simulink model "Merge_Tryout"  (R2020b)
settings: Solver=VariableStepAuto  StartTime=0.0  StopTime=60  RelTol=1e-3
values from neighbouring files (symbols this model uses):
  A_2 = zeros(3)    [MPC_tune.m]
  B_2 = I_inv    [MPC_tune.m]
  C_2 = eye(3)    [MPC_tune.m]
  D_2 = zeros(3)    [MPC_tune.m]
  I_inv = inv(I_mat)    [MPC_tune.m]
undefined symbols (not defined in the file or in its folder): theta0, x0
libraries: fuzblock x6, pid_lib x3, mpclib x2, dspmathops x2, dspsigops x2
settings Model: Creator=Jonathan van Zyl  LastModifiedBy=Jonathan van Zyl

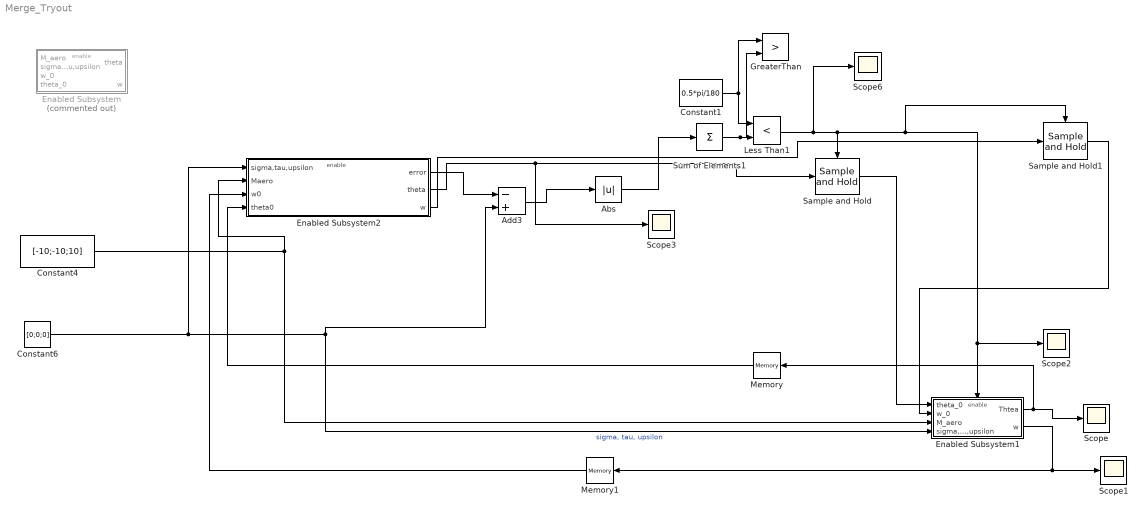
== system Merge_Tryout ==
  Abs : Abs
  Add3 : Sum  Inputs=-+
  Constant1 : Constant  Value=0.5*pi/180
  Constant4 : Constant  Value=[-10;-10;10]
  Constant6 : Constant  Value=[0;0;0]
  Enabled Subsystem : Subsystem  Commented=on  TreatAsAtomicUnit=on
  Enabled Subsystem1 : Subsystem  TreatAsAtomicUnit=on
  Enabled Subsystem2 : Subsystem  TreatAsAtomicUnit=on
  GreaterThan : RelationalOperator  Operator=>  OutDataTypeStr=boolean  RndMeth=Simplest
  Less Than1 : RelationalOperator  Operator=<  OutDataTypeStr=boolean  RndMeth=Simplest
  Memory : Memory
  Memory1 : Memory
  Sample and Hold : dspsigops/Sample and Hold  trig=Rising edge  initCond=0  latchinput=off
  Sample and Hold1 : dspsigops/Sample and Hold  trig=Rising edge  initCond=0  latchinput=off
  Scope{,1..3,6} (5 alike) : Scope
  Sum of Elements1 : Sum  Inputs=+
  wires:
  Constant4/1 -> Enabled Subsystem2/2(Maero), Enabled Subsystem1/3(M_aero)
  Constant6/1 -> Add3/2, Enabled Subsystem1/4(sigma,tau,upsilon), Enabled Subsystem2/1(sigma,tau,upsilon)  "sigma, tau, upsilon"
  Add3/1 -> Abs/1
  Less Than1/1 -> Scope2/1, Enabled Subsystem1/Enable, Sample and Hold1/Trigger, Sample and Hold/Trigger, Scope6/1
  Sum of Elements1/1 -> GreaterThan/2, Less Than1/2
  Constant1/1 -> GreaterThan/1, Less Than1/1
  Abs/1 -> Sum of Elements1/1
  Sample and Hold/1 -> Enabled Subsystem1/1(theta_0)
  Sample and Hold1/1 -> Enabled Subsystem1/2(w_0)
  Enabled Subsystem2/1(error) -> Add3/1
  ? -> Enabled Subsystem2/Enable
  Enabled Subsystem1/1(Thtea) -> Memory/1, Scope/1
  Enabled Subsystem2/2(theta) -> Scope3/1, Sample and Hold/1
  Enabled Subsystem2/3(w) -> Sample and Hold1/1
  Memory/1 -> Enabled Subsystem2/4(theta0)
  Enabled Subsystem1/2(w) -> Memory1/1, Scope1/1
  Memory1/1 -> Enabled Subsystem2/3(w0)

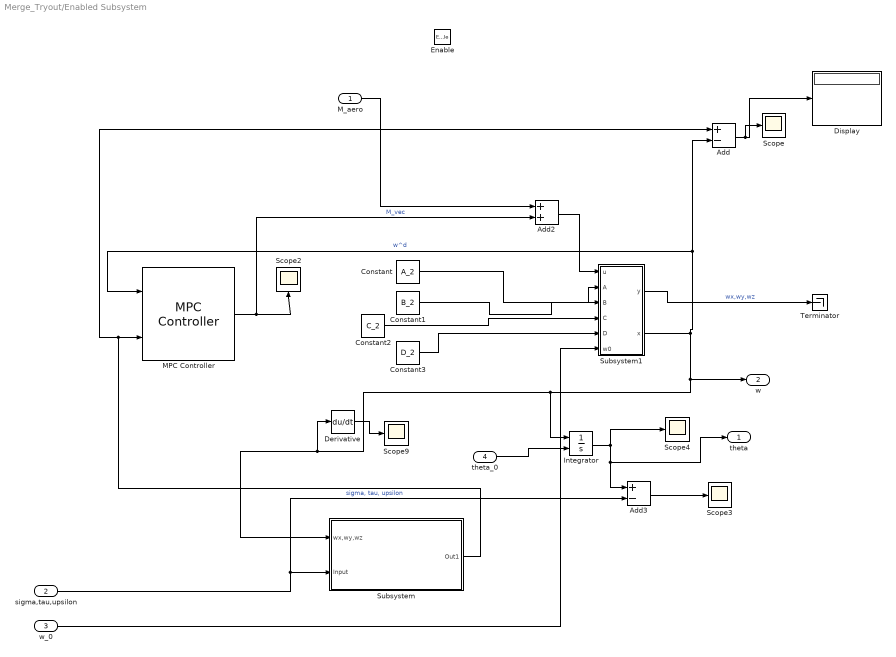
== system Merge_Tryout/Enabled Subsystem ==
  M_aero : Inport
  sigma,tau,upsilon : Inport  Port=2
  w_0 : Inport  Port=3
  theta_0 : Inport  Port=4
  Enable : EnablePort
  Add : Sum  Inputs=+-
  Add2 : Sum
  Add3 : Sum  Inputs=+-
  Constant : Constant  Value=A_2
  Constant1 : Constant  Value=B_2
  Constant2 : Constant  Value=C_2
  Constant3 : Constant  Value=D_2
  Derivative : Derivative
  Display : Display
  Integrator : Integrator  InitialConditionSource=external
  MPC Controller : mpclib/MPC Controller  SCDEnableBlockLinearizationSpecification=on  mpcobj=MPCDesignerSession.AppData.Controllers.MPC  is_multiple=0  enable_value=0  return_u0=off  updateMPCinCallerWorkspace=on  md_inport=off  mv_inport=off  uref_inport=off  return_cost=off  return_mvseq=off  return_qpstatus=off  return_xseq=off  return_state=off  return_ovseq=off  state_inport=off  umin_inport=off  umax_inport=off  ymin_inport=off  ymax_inport=off  cc_inport=off  ywt_inport=off  uwt_inport=off  duwt_inport=off  rhoeps_inport=off  pm_inport=off  MaximumP=10  HorizonChoice=FixedHorizon  n_ts=0.1  n_p=10  n_mv=3  n_md=0  n_ud=0  n_mo=3  n_uo=0  BlockDataType=double  SampleTimeInherited=off  switch_inport=off
  Scope{,2..4,9} (5 alike) : Scope
  Subsystem : Subsystem
  Subsystem1 : Subsystem
  Terminator : Terminator
  theta : Outport
  w : Outport  Port=2
  wires:
  Constant2/1 -> Subsystem1/4(C)
  Subsystem1/2(x) -> Add/2, MPC Controller/1, w/1, Integrator/1, Subsystem/1(wx,wy,wz), Derivative/1  "w^d"
  Derivative/1 -> Scope9/1
  MPC Controller/1 -> Add2/2, Scope2/1  "M_vec"
  Constant3/1 -> Subsystem1/5(D)
  sigma,tau,upsilon/1 -> Add3/2, Subsystem/2(Input)  "sigma, tau, upsilon"
  Subsystem/1(Out1) -> Add/1, MPC Controller/2
  M_aero/1 -> Add2/1
  Add/1 -> Display/1, Scope/1
  Constant/1 -> Subsystem1/2(A)
  Add2/1 -> Subsystem1/1(u)
  Add3/1 -> Scope3/1
  Subsystem1/1(y) -> Terminator/1  "wx,wy,wz"
  Constant1/1 -> Subsystem1/3(B)
  Integrator/1 -> Scope4/1, Add3/1, theta/1
  w_0/1 -> Subsystem1/6(w0)
  theta_0/1 -> Integrator/2

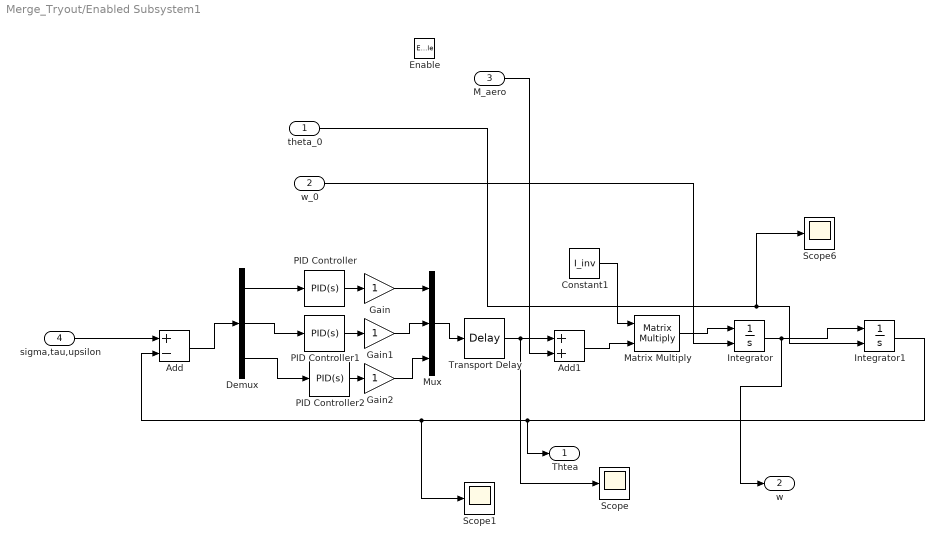
== system Merge_Tryout/Enabled Subsystem1 ==
  theta_0 : Inport
  w_0 : Inport  Port=2
  M_aero : Inport  Port=3
  sigma,tau,upsilon : Inport  Port=4
  Enable : EnablePort
  Add : Sum  Inputs=+-
  Add1 : Sum
  Constant1 : Constant  Value=I_inv
  Demux : Demux  Outputs=3
  Gain : Gain
  Gain1 : Gain
  Gain2 : Gain
  Integrator : Integrator  InitialConditionSource=external  InitialCondition=[0.15;-0.2;0.01]
  Integrator1 : Integrator  InitialConditionSource=external  InitialCondition=[0.01;-0.01;0.005]
  Matrix Multiply : Product  Multiplication=Matrix(*)
  Mux : Mux  Inputs=3
  PID Controller : pid_lib/PID Controller  Controller=PID  Form=Parallel  TimeDomain=Continuous-time  UseExternalTs=off  SampleTime=-1  IntegratorMethod=Forward Euler  FilterMethod=Forward Euler  ControllerParametersSource=internal  P=76.4274415550338  I=3.57793373088927  D=400.875615235633  UseFilter=on  N=5.45397025421619  TunerSelectOption=Transfer Function Based (PID Tuner App)  InitialConditionSource=internal  InitialConditionForIntegrator=0  InitialConditionForFilter=0  DifferentiatorICPrevScaledInput=0  ExternalReset=none  TrackingMode=off  Kt=1  LimitOutput=off  SatLimitsSource=internal  UpperSaturationLimit=inf  LowerSaturationLimit=-inf  LinearizeAsGain=on  AntiWindupMode=none  Kb=1  POutMin=[]  POutMax=[]  IOutMin=[]  IOutMax=[]  DOutMin=[]  DOutMax=[]  NOutMin=[]  NOutMax=[]  SumOutMin=[]  SumOutMax=[]  SaturationOutMin=[]  SaturationOutMax=[]  PParamMin=[]  PParamMax=[]  IParamMin=[]  IParamMax=[]  DParamMin=[]  DParamMax=[]  NParamMin=[]  NParamMax=[]  KbParamMin=[]  KbParamMax=[]  KtParamMin=[]  KtParamMax=[]  KbOutMin=[]  KbOutMax=[]  KtOutMin=[]  KtOutMax=[]  IntegratorOutMin=[]  IntegratorOutMax=[]  FilterOutMin=[]  FilterOutMax=[]  SumI1OutMin=[]  SumI1OutMax=[]  SumI2OutMin=[]  SumI2OutMax=[]  SumI3OutMin=[]  SumI3OutMax=[]  SumI4OutMin=[]  SumI4OutMax=[]  SumDOutMin=[]  SumDOutMax=[]  DifferentiatorOutMin=[]  DifferentiatorOutMax=[]  FilterDiffOutCoefMin=[]  FilterDiffOutCoefMax=[]  ReciprocalOutMin=[]  ReciprocalOutMax=[]  SumDenOutMin=[]  SumDenOutMax=[]  SumNumOutMin=[]  SumNumOutMax=[]  DivideOutMin=[]  DivideOutMax=[]  UdiffTsProdOutMin=[]  UdiffTsProdOutMax=[]  NTsProdOutMin=[]  NTsProdOutMax=[]  UintegralTsProdOutMin=[]  UintegralTsProdOutMax=[]  UngainTsProdOutMin=[]  UngainTsProdOutMax=[]  IntegratorContinuousStateAttributes=''  IntegratorStateMustResolveToSignalObject=off  IntegratorRTWStateStorageClass=Auto  FilterContinuousStateAttributes=''  FilterStateMustResolveToSignalObject=off  FilterRTWStateStorageClass=Auto  ParallelPVariant=InternalParameters  IdealPVariant=Disabled  IVariant=InternalParameters  DVariant=InternalParameters  IntegratorVariant=Continuous  SatVariant=Disabled  AWVariant=Passthrough  PCopyVariant=Disabled  TRVariant=Disabled  FdbkBlocksVariant=Forward  IdealPFdbkVariant=Disabled  SatFdbkVariant=Disabled  DerivativeFilterVariant=ContFilter  NVariant=InternalParameters  NCopyVariant=Disabled  FilterICVariant=InternalICsFilter  IntegratorICVariant=InternalICs  ExternalResetVariant=Disabled  TRSumVariant=Passthrough  SumFdbkVariant=Disabled  SumVariant=Sum_PID  TsampFilterVariant=InternalTs  TsampNgainVariant=Passthrough  TsampIntegralVariant=Passthrough  ExternalSaturationOutDataTypeStr=Inherit: Same as second input
  PID Controller1 : pid_lib/PID Controller  Controller=PID  Form=Parallel  TimeDomain=Continuous-time  UseExternalTs=off  SampleTime=-1  IntegratorMethod=Forward Euler  FilterMethod=Forward Euler  ControllerParametersSource=internal  P=-202.527799620363  I=-9.48129403471772  D=-1062.29457146841  UseFilter=on  N=5.45397025421619  TunerSelectOption=Transfer Function Based (PID Tuner App)  InitialConditionSource=internal  InitialConditionForIntegrator=0  InitialConditionForFilter=0  DifferentiatorICPrevScaledInput=0  ExternalReset=none  TrackingMode=off  Kt=1  LimitOutput=off  SatLimitsSource=internal  UpperSaturationLimit=inf  LowerSaturationLimit=-inf  LinearizeAsGain=on  AntiWindupMode=none  Kb=1  POutMin=[]  POutMax=[]  IOutMin=[]  IOutMax=[]  DOutMin=[]  DOutMax=[]  NOutMin=[]  NOutMax=[]  SumOutMin=[]  SumOutMax=[]  SaturationOutMin=[]  SaturationOutMax=[]  PParamMin=[]  PParamMax=[]  IParamMin=[]  IParamMax=[]  DParamMin=[]  DParamMax=[]  NParamMin=[]  NParamMax=[]  KbParamMin=[]  KbParamMax=[]  KtParamMin=[]  KtParamMax=[]  KbOutMin=[]  KbOutMax=[]  KtOutMin=[]  KtOutMax=[]  IntegratorOutMin=[]  IntegratorOutMax=[]  FilterOutMin=[]  FilterOutMax=[]  SumI1OutMin=[]  SumI1OutMax=[]  SumI2OutMin=[]  SumI2OutMax=[]  SumI3OutMin=[]  SumI3OutMax=[]  SumI4OutMin=[]  SumI4OutMax=[]  SumDOutMin=[]  SumDOutMax=[]  DifferentiatorOutMin=[]  DifferentiatorOutMax=[]  FilterDiffOutCoefMin=[]  FilterDiffOutCoefMax=[]  ReciprocalOutMin=[]  ReciprocalOutMax=[]  SumDenOutMin=[]  SumDenOutMax=[]  SumNumOutMin=[]  SumNumOutMax=[]  DivideOutMin=[]  DivideOutMax=[]  UdiffTsProdOutMin=[]  UdiffTsProdOutMax=[]  NTsProdOutMin=[]  NTsProdOutMax=[]  UintegralTsProdOutMin=[]  UintegralTsProdOutMax=[]  UngainTsProdOutMin=[]  UngainTsProdOutMax=[]  IntegratorContinuousStateAttributes=''  IntegratorStateMustResolveToSignalObject=off  IntegratorRTWStateStorageClass=Auto  FilterContinuousStateAttributes=''  FilterStateMustResolveToSignalObject=off  FilterRTWStateStorageClass=Auto  ParallelPVariant=InternalParameters  IdealPVariant=Disabled  IVariant=InternalParameters  DVariant=InternalParameters  IntegratorVariant=Continuous  SatVariant=Disabled  AWVariant=Passthrough  PCopyVariant=Disabled  TRVariant=Disabled  FdbkBlocksVariant=Forward  IdealPFdbkVariant=Disabled  SatFdbkVariant=Disabled  DerivativeFilterVariant=ContFilter  NVariant=InternalParameters  NCopyVariant=Disabled  FilterICVariant=InternalICsFilter  IntegratorICVariant=InternalICs  ExternalResetVariant=Disabled  TRSumVariant=Passthrough  SumFdbkVariant=Disabled  SumVariant=Sum_PID  TsampFilterVariant=InternalTs  TsampNgainVariant=Passthrough  TsampIntegralVariant=Passthrough  ExternalSaturationOutDataTypeStr=Inherit: Same as second input
  PID Controller2 : pid_lib/PID Controller  Controller=PID  Form=Parallel  TimeDomain=Continuous-time  UseExternalTs=off  SampleTime=-1  IntegratorMethod=Forward Euler  FilterMethod=Forward Euler  ControllerParametersSource=internal  P=-232.294042315359  I=-10.8747940867059  D=-1218.42384402842  UseFilter=on  N=5.45397025421619  TunerSelectOption=Transfer Function Based (PID Tuner App)  InitialConditionSource=internal  InitialConditionForIntegrator=0  InitialConditionForFilter=0  DifferentiatorICPrevScaledInput=0  ExternalReset=none  TrackingMode=off  Kt=1  LimitOutput=off  SatLimitsSource=internal  UpperSaturationLimit=inf  LowerSaturationLimit=-inf  LinearizeAsGain=on  AntiWindupMode=none  Kb=1  POutMin=[]  POutMax=[]  IOutMin=[]  IOutMax=[]  DOutMin=[]  DOutMax=[]  NOutMin=[]  NOutMax=[]  SumOutMin=[]  SumOutMax=[]  SaturationOutMin=[]  SaturationOutMax=[]  PParamMin=[]  PParamMax=[]  IParamMin=[]  IParamMax=[]  DParamMin=[]  DParamMax=[]  NParamMin=[]  NParamMax=[]  KbParamMin=[]  KbParamMax=[]  KtParamMin=[]  KtParamMax=[]  KbOutMin=[]  KbOutMax=[]  KtOutMin=[]  KtOutMax=[]  IntegratorOutMin=[]  IntegratorOutMax=[]  FilterOutMin=[]  FilterOutMax=[]  SumI1OutMin=[]  SumI1OutMax=[]  SumI2OutMin=[]  SumI2OutMax=[]  SumI3OutMin=[]  SumI3OutMax=[]  SumI4OutMin=[]  SumI4OutMax=[]  SumDOutMin=[]  SumDOutMax=[]  DifferentiatorOutMin=[]  DifferentiatorOutMax=[]  FilterDiffOutCoefMin=[]  FilterDiffOutCoefMax=[]  ReciprocalOutMin=[]  ReciprocalOutMax=[]  SumDenOutMin=[]  SumDenOutMax=[]  SumNumOutMin=[]  SumNumOutMax=[]  DivideOutMin=[]  DivideOutMax=[]  UdiffTsProdOutMin=[]  UdiffTsProdOutMax=[]  NTsProdOutMin=[]  NTsProdOutMax=[]  UintegralTsProdOutMin=[]  UintegralTsProdOutMax=[]  UngainTsProdOutMin=[]  UngainTsProdOutMax=[]  IntegratorContinuousStateAttributes=''  IntegratorStateMustResolveToSignalObject=off  IntegratorRTWStateStorageClass=Auto  FilterContinuousStateAttributes=''  FilterStateMustResolveToSignalObject=off  FilterRTWStateStorageClass=Auto  ParallelPVariant=InternalParameters  IdealPVariant=Disabled  IVariant=InternalParameters  DVariant=InternalParameters  IntegratorVariant=Continuous  SatVariant=Disabled  AWVariant=Passthrough  PCopyVariant=Disabled  TRVariant=Disabled  FdbkBlocksVariant=Forward  IdealPFdbkVariant=Disabled  SatFdbkVariant=Disabled  DerivativeFilterVariant=ContFilter  NVariant=InternalParameters  NCopyVariant=Disabled  FilterICVariant=InternalICsFilter  IntegratorICVariant=InternalICs  ExternalResetVariant=Disabled  TRSumVariant=Passthrough  SumFdbkVariant=Disabled  SumVariant=Sum_PID  TsampFilterVariant=InternalTs  TsampNgainVariant=Passthrough  TsampIntegralVariant=Passthrough  ExternalSaturationOutDataTypeStr=Inherit: Same as second input
  Scope : Scope
  Scope1 : Scope
  Scope6 : Scope
  Transport Delay : TransportDelay  DelayTime=0.1
  Thtea : Outport
  w : Outport  Port=2
  wires:
  Demux/1 -> PID Controller/1
  Gain/1 -> Mux/1
  PID Controller1/1 -> Gain1/1
  Mux/1 -> Transport Delay/1
  theta_0/1 -> Integrator1/2, Scope6/1
  Demux/2 -> PID Controller1/1
  Constant1/1 -> Matrix Multiply/1
  Demux/3 -> PID Controller2/1
  sigma,tau,upsilon/1 -> Add/1
  Integrator1/1 -> Thtea/1, Scope1/1, Add/2
  Gain2/1 -> Mux/3
  Add/1 -> Demux/1
  Matrix Multiply/1 -> Integrator/1
  PID Controller2/1 -> Gain2/1
  Gain1/1 -> Mux/2
  Integrator/1 -> w/1, Integrator1/1
  PID Controller/1 -> Gain/1
  w_0/1 -> Integrator/2
  M_aero/1 -> Add1/2
  Add1/1 -> Matrix Multiply/2
  Transport Delay/1 -> Scope/1, Add1/1

== system Merge_Tryout/Enabled Subsystem2 ==
  sigma,tau,upsilon : Inport
  Maero : Inport  Port=2
  w0 : Inport  Port=3
  theta0 : Inport  Port=4
  Enable : EnablePort
  Add : Sum  Inputs=-+
  Subsystem : Subsystem
  error : Outport
  theta : Outport  Port=2
  w : Outport  Port=3
  wires:
  Subsystem/1(theta) -> theta/1, Add/1
  Add/1 -> error/1
  Maero/1 -> Subsystem/1(M_aero)
  sigma,tau,upsilon/1 -> Add/2, Subsystem/2(sigma,tau,upsilon)  "sigma, tau, upsilon"
  Subsystem/2(w) -> w/1
  w0/1 -> Subsystem/3(w0)
  theta0/1 -> Subsystem/4(tehat0)

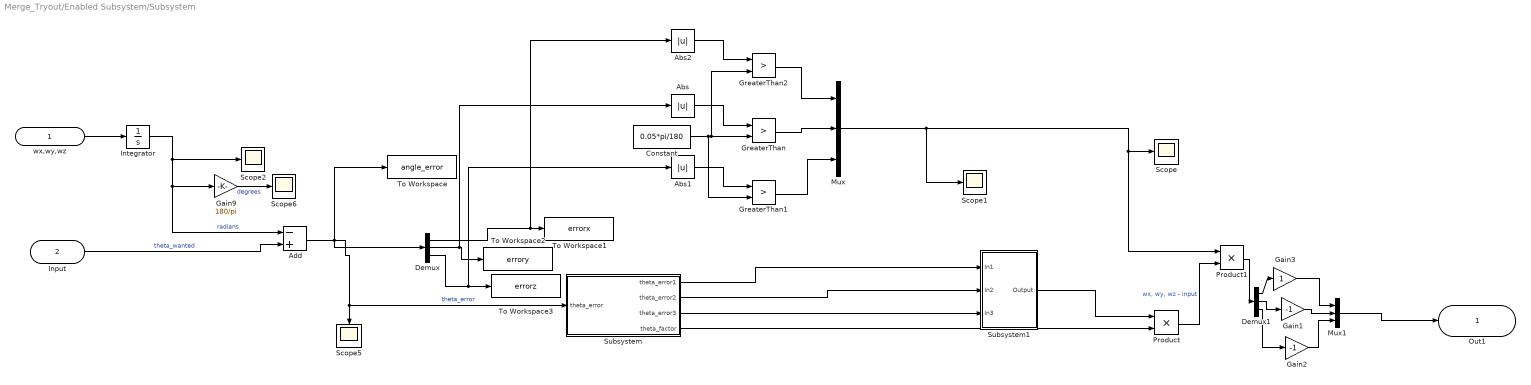
== system Merge_Tryout/Enabled Subsystem/Subsystem ==
  wx,wy,wz : Inport
  Input : Inport  Port=2
  Abs : Abs
  Abs1 : Abs
  Abs2 : Abs
  Add : Sum  Inputs=-+
  Constant : Constant  Value=0.05*pi/180
  Demux : Demux  Outputs=3
  Demux1 : Demux  Outputs=3
  Gain1 : Gain  Gain=-1
  Gain2 : Gain  Gain=-1
  Gain3 : Gain
  Gain9 : Gain  Gain=180/pi
  GreaterThan : RelationalOperator  Operator=>  OutDataTypeStr=boolean  RndMeth=Simplest
  GreaterThan1 : RelationalOperator  Operator=>  OutDataTypeStr=boolean  RndMeth=Simplest
  GreaterThan2 : RelationalOperator  Operator=>  OutDataTypeStr=boolean  RndMeth=Simplest
  Integrator : Integrator  InitialCondition=[0;0;0]
  Mux : Mux  Inputs=3
  Mux1 : Mux  Inputs=3
  Product : Product
  Product1 : Product
  Scope{,1..2,5..6} (5 alike) : Scope
  Subsystem : Subsystem
  Subsystem1 : Subsystem
  To Workspace : ToWorkspace  VariableName=angle_error  SampleTime=-1
  To Workspace1 : ToWorkspace  VariableName=errorx  SaveFormat=Timeseries  SampleTime=-1
      settings: Save2DSignal=2-D array (concatenate along first dimension)
  To Workspace2 : ToWorkspace  VariableName=errory  SaveFormat=Timeseries  SampleTime=-1
  To Workspace3 : ToWorkspace  VariableName=errorz  SaveFormat=Timeseries  SampleTime=-1
  Out1 : Outport
  wires:
  Integrator/1 -> Add/1, Gain9/1, Scope2/1  "radians"
  Add/1 -> To Workspace/1, Demux/1, Subsystem/1(theta_error), Scope5/1  "theta_error"
  Gain9/1 -> Scope6/1  "degrees"
  Input/1 -> Add/2  "theta_wanted"
  Product/1 -> Product1/2  "wx, wy, wz - input"
  wx,wy,wz/1 -> Integrator/1
  Subsystem/4(theta_factor) -> Product/2
  Demux/2 -> Abs/1, To Workspace2/1
  Demux/3 -> Abs1/1, To Workspace3/1
  Demux/1 -> Abs2/1, To Workspace1/1
  Subsystem/1(theta_error1) -> Subsystem1/1(In1)
  Subsystem/2(theta_error2) -> Subsystem1/2(In2)
  Subsystem/3(theta_error3) -> Subsystem1/3(In3)
  Subsystem1/1(Output) -> Product/1
  Abs/1 -> GreaterThan/1
  Constant/1 -> GreaterThan1/2, GreaterThan2/2, GreaterThan/2
  Abs1/1 -> GreaterThan1/1
  Abs2/1 -> GreaterThan2/1
  GreaterThan2/1 -> Mux/1
  GreaterThan/1 -> Mux/2
  GreaterThan1/1 -> Mux/3
  Mux/1 -> Scope1/1, Scope/1, Product1/1
  Product1/1 -> Demux1/1
  Mux1/1 -> Out1/1
  Demux1/2 -> Gain1/1
  Demux1/3 -> Gain2/1
  Demux1/1 -> Gain3/1
  Gain3/1 -> Mux1/1
  Gain1/1 -> Mux1/2
  Gain2/1 -> Mux1/3

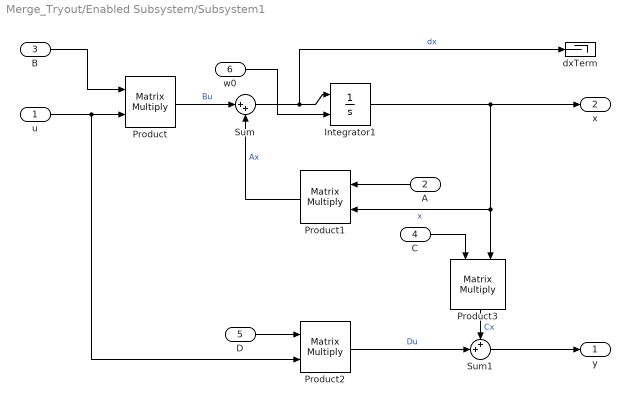
== system Merge_Tryout/Enabled Subsystem/Subsystem1 ==
  u : Inport
  A : Inport  Port=2
  B : Inport  Port=3
  C : Inport  Port=4
  D : Inport  Port=5
  w0 : Inport  Port=6
  Integrator1 : Integrator  InitialConditionSource=external  InitialCondition=x0
  Product{,1..3} (4 alike) : Product  SCDEnableBlockLinearizationSpecification=on  Multiplication=Matrix(*)
  Sum : Sum  Inputs=|++
  Sum1 : Sum  Inputs=++|
  dxTerm : Terminator
  y : Outport  VectorParamsAs1DForOutWhenUnconnected=off
  x : Outport  Port=2  VectorParamsAs1DForOutWhenUnconnected=off
  wires:
  Sum/1 -> Integrator1/1, dxTerm/1  "dx"
  Product3/1 -> Sum1/1  "Cx"
  Product/1 -> Sum/1  "Bu"
  u/1 -> Product2/2, Product/2
  Product2/1 -> Sum1/2  "Du"
  Integrator1/1 -> x/1, Product1/2, Product3/2  "x"
  A/1 -> Product1/1
  Product1/1 -> Sum/2  "Ax"
  C/1 -> Product3/1
  B/1 -> Product/1
  D/1 -> Product2/1
  Sum1/1 -> y/1
  w0/1 -> Integrator1/2

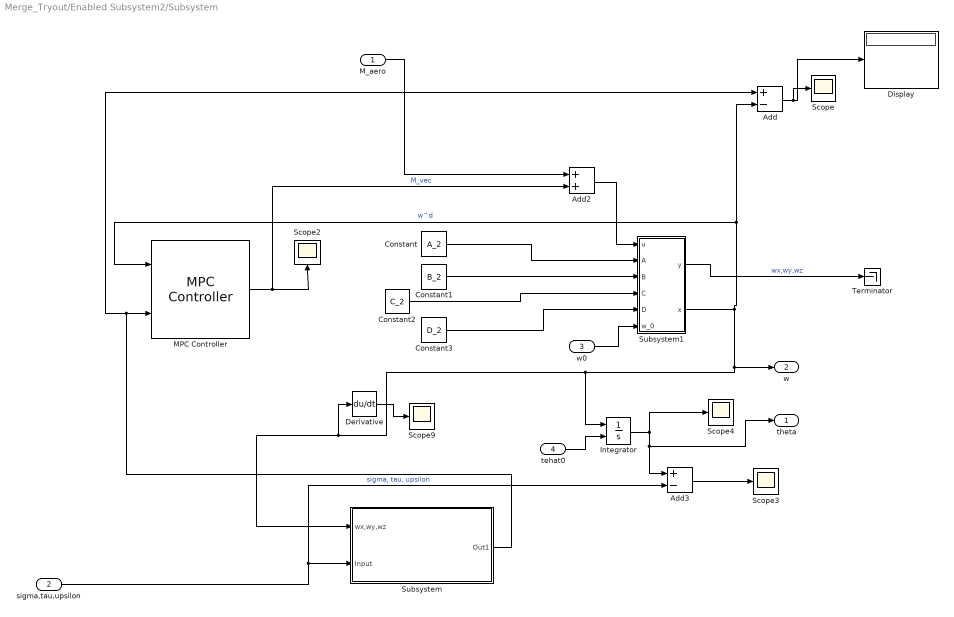
== system Merge_Tryout/Enabled Subsystem2/Subsystem ==
  M_aero : Inport
  sigma,tau,upsilon : Inport  Port=2
  w0 : Inport  Port=3
  tehat0 : Inport  Port=4
  Add : Sum  Inputs=+-
  Add2 : Sum
  Add3 : Sum  Inputs=+-
  Constant : Constant  Value=A_2
  Constant1 : Constant  Value=B_2
  Constant2 : Constant  Value=C_2
  Constant3 : Constant  Value=D_2
  Derivative : Derivative
  Display : Display
  Integrator : Integrator  InitialConditionSource=external  InitialCondition=theta0
  MPC Controller : mpclib/MPC Controller  SCDEnableBlockLinearizationSpecification=on  mpcobj=MPCDesignerSession.AppData.Controllers.MPC  is_multiple=0  enable_value=0  return_u0=off  updateMPCinCallerWorkspace=on  md_inport=off  mv_inport=off  uref_inport=off  return_cost=off  return_mvseq=off  return_qpstatus=off  return_xseq=off  return_state=off  return_ovseq=off  state_inport=off  umin_inport=off  umax_inport=off  ymin_inport=off  ymax_inport=off  cc_inport=off  ywt_inport=off  uwt_inport=off  duwt_inport=off  rhoeps_inport=off  pm_inport=off  MaximumP=10  HorizonChoice=FixedHorizon  n_ts=0.1  n_p=10  n_mv=3  n_md=0  n_ud=0  n_mo=3  n_uo=0  BlockDataType=double  SampleTimeInherited=off  switch_inport=off
  Scope{,2..4,9} (5 alike) : Scope
  Subsystem : Subsystem
  Subsystem1 : Subsystem
  Terminator : Terminator
  theta : Outport
  w : Outport  Port=2
  wires:
  Subsystem1/1(y) -> Terminator/1  "wx,wy,wz"
  Derivative/1 -> Scope9/1
  Integrator/1 -> Scope4/1, Add3/1, theta/1
  Add/1 -> Display/1, Scope/1
  Add3/1 -> Scope3/1
  Add2/1 -> Subsystem1/1(u)
  sigma,tau,upsilon/1 -> Add3/2, Subsystem/2(Input)  "sigma, tau, upsilon"
  Subsystem/1(Out1) -> Add/1, MPC Controller/2
  M_aero/1 -> Add2/1
  Constant2/1 -> Subsystem1/4(C)
  Constant3/1 -> Subsystem1/5(D)
  Subsystem1/2(x) -> Add/2, MPC Controller/1, w/1, Integrator/1, Subsystem/1(wx,wy,wz), Derivative/1  "w^d"
  MPC Controller/1 -> Add2/2, Scope2/1  "M_vec"
  Constant/1 -> Subsystem1/2(A)
  Constant1/1 -> Subsystem1/3(B)
  w0/1 -> Subsystem1/6(w_0)
  tehat0/1 -> Integrator/2

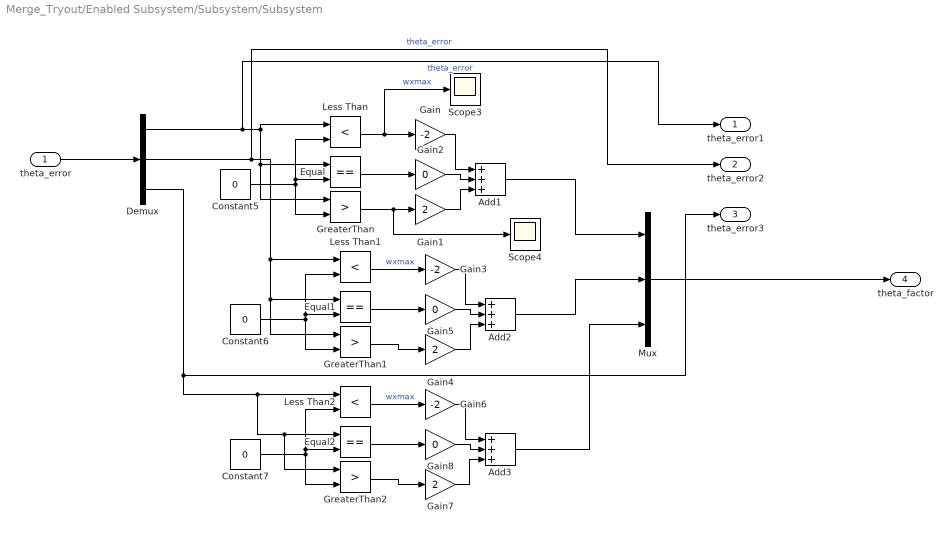
== system Merge_Tryout/Enabled Subsystem/Subsystem/Subsystem ==
  theta_error : Inport
  Add1 : Sum  Inputs=+++
  Add2 : Sum  Inputs=+++
  Add3 : Sum  Inputs=+++
  Constant5 : Constant  Value=0
  Constant6 : Constant  Value=0
  Constant7 : Constant  Value=0
  Demux : Demux  Outputs=3
  Equal : RelationalOperator  Operator===  OutDataTypeStr=boolean  RndMeth=Simplest
  Equal1 : RelationalOperator  Operator===  OutDataTypeStr=boolean  RndMeth=Simplest
  Equal2 : RelationalOperator  Operator===  OutDataTypeStr=boolean  RndMeth=Simplest
  Gain : Gain  Gain=-2
  Gain1 : Gain  Gain=2
  Gain2 : Gain  Gain=0
  Gain3 : Gain  Gain=-2
  Gain4 : Gain  Gain=2
  Gain5 : Gain  Gain=0
  Gain6 : Gain  Gain=-2
  Gain7 : Gain  Gain=2
  Gain8 : Gain  Gain=0
  GreaterThan : RelationalOperator  Operator=>  OutDataTypeStr=boolean  RndMeth=Simplest
  GreaterThan1 : RelationalOperator  Operator=>  OutDataTypeStr=boolean  RndMeth=Simplest
  GreaterThan2 : RelationalOperator  Operator=>  OutDataTypeStr=boolean  RndMeth=Simplest
  Less Than : RelationalOperator  Operator=<  OutDataTypeStr=boolean  RndMeth=Simplest
  Less Than1 : RelationalOperator  Operator=<  OutDataTypeStr=boolean  RndMeth=Simplest
  Less Than2 : RelationalOperator  Operator=<  OutDataTypeStr=boolean  RndMeth=Simplest
  Mux : Mux  Inputs=3
  Scope3 : Scope
  Scope4 : Scope
  theta_error1 : Outport
  theta_error2 : Outport  Port=2
  theta_error3 : Outport  Port=3
  theta_factor : Outport  Port=4
  wires:
  Add1/1 -> Mux/1
  Constant5/1 -> Equal/2, Less Than/2, GreaterThan/2
  Equal2/1 -> Gain8/1
  Demux/1 -> theta_error1/1, GreaterThan/1, Equal/1, Less Than/1  "theta_error"
  GreaterThan2/1 -> Gain7/1
  Gain1/1 -> Add1/3
  Gain7/1 -> Add3/3
  Less Than1/1 -> Gain3/1  "wxmax"
  Gain6/1 -> Add3/1
  Equal/1 -> Gain2/1
  Gain5/1 -> Add2/2
  Add3/1 -> Mux/3
  GreaterThan/1 -> Scope4/1, Gain1/1
  Constant6/1 -> Equal1/2, Less Than1/2, GreaterThan1/2
  Demux/3 -> theta_error3/1, GreaterThan2/1, Equal2/1, Less Than2/1
  Gain3/1 -> Add2/1
  Constant7/1 -> Equal2/2, Less Than2/2, GreaterThan2/2
  Equal1/1 -> Gain5/1
  Gain8/1 -> Add3/2
  Gain4/1 -> Add2/3
  GreaterThan1/1 -> Gain4/1
  Gain/1 -> Add1/1
  Demux/2 -> theta_error2/1, GreaterThan1/1, Equal1/1, Less Than1/1  "theta_error"
  Gain2/1 -> Add1/2
  Add2/1 -> Mux/2
  Less Than/1 -> Scope3/1, Gain/1  "wxmax"
  Less Than2/1 -> Gain6/1  "wxmax"
  theta_error/1 -> Demux/1
  Mux/1 -> theta_factor/1

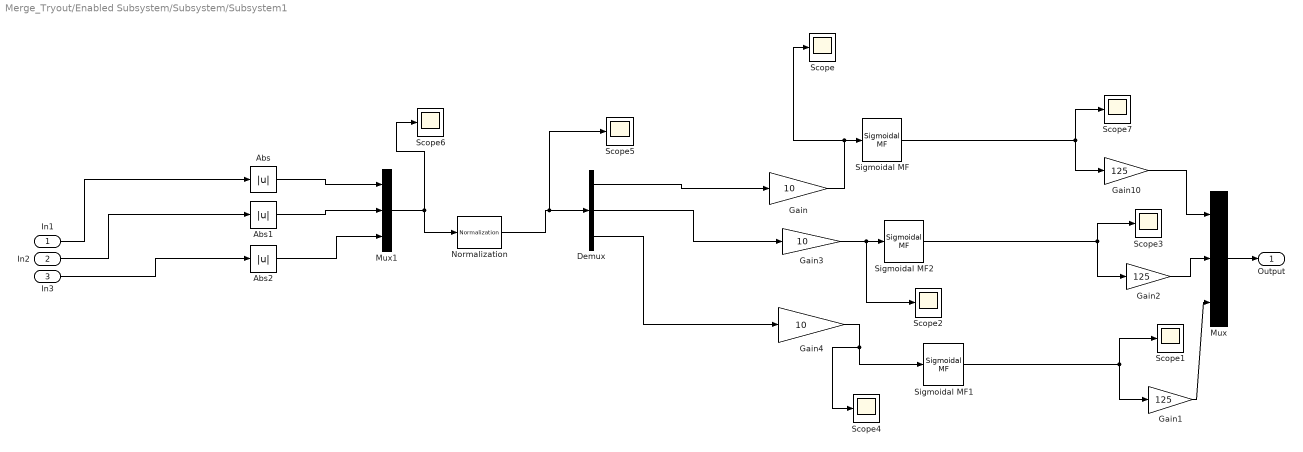
== system Merge_Tryout/Enabled Subsystem/Subsystem/Subsystem1 ==
  In1 : Inport
  In2 : Inport  Port=2
  In3 : Inport  Port=3
  Abs : Abs
  Abs1 : Abs
  Abs2 : Abs
  Demux : Demux  Outputs=3
  Gain : Gain  Gain=10
  Gain1 : Gain  Gain=125
  Gain10 : Gain  Gain=125
  Gain2 : Gain  Gain=125
  Gain3 : Gain  Gain=10
  Gain4 : Gain  Gain=10
  Mux : Mux  Inputs=3
  Mux1 : Mux  Inputs=3
  Normalization : dspmathops/Normalization  NormType=Squared 2-norm  Bias=1e-10  NormOver=Each column  Dimension=1  roundingMode=Floor  overflowMode=off  accumDataTypeStr=Inherit: Same as product output  accumLastDataTypeStr=Inherit: Same as product output  outputDataTypeStr=Inherit: Same as product output  outputMin=[]  outputMax=[]  outputLastDataTypeStr=Inherit: Same as product output
  Scope{,1..7} (8 alike) : Scope
  Sigmoidal MF : fuzblock/Membership  Functions/Sigmoidal MF  a=10^(-8)  c=1000
      settings: SourceProductBaseCode=FL
  Sigmoidal MF1 : fuzblock/Membership  Functions/Sigmoidal MF  a=10^(-8)  c=1000
      settings: SourceProductBaseCode=FL
  Sigmoidal MF2 : fuzblock/Membership  Functions/Sigmoidal MF  a=10^(-8)  c=1000
      settings: SourceProductBaseCode=FL
  Output : Outport
  wires:
  Gain2/1 -> Mux/2
  Gain10/1 -> Mux/1
  Sigmoidal MF1/1 -> Gain1/1, Scope1/1
  Sigmoidal MF/1 -> Gain10/1, Scope7/1
  Sigmoidal MF2/1 -> Gain2/1, Scope3/1
  Gain/1 -> Scope/1, Sigmoidal MF/1
  Gain1/1 -> Mux/3
  Gain3/1 -> Scope2/1, Sigmoidal MF2/1
  In2/1 -> Abs1/1
  In1/1 -> Abs/1
  In3/1 -> Abs2/1
  Mux/1 -> Output/1
  Abs/1 -> Mux1/1
  Abs1/1 -> Mux1/2
  Gain4/1 -> Scope4/1, Sigmoidal MF1/1
  Abs2/1 -> Mux1/3
  Demux/3 -> Gain4/1
  Demux/1 -> Gain/1
  Demux/2 -> Gain3/1
  Mux1/1 -> Normalization/1, Scope6/1
  Normalization/1 -> Scope5/1, Demux/1

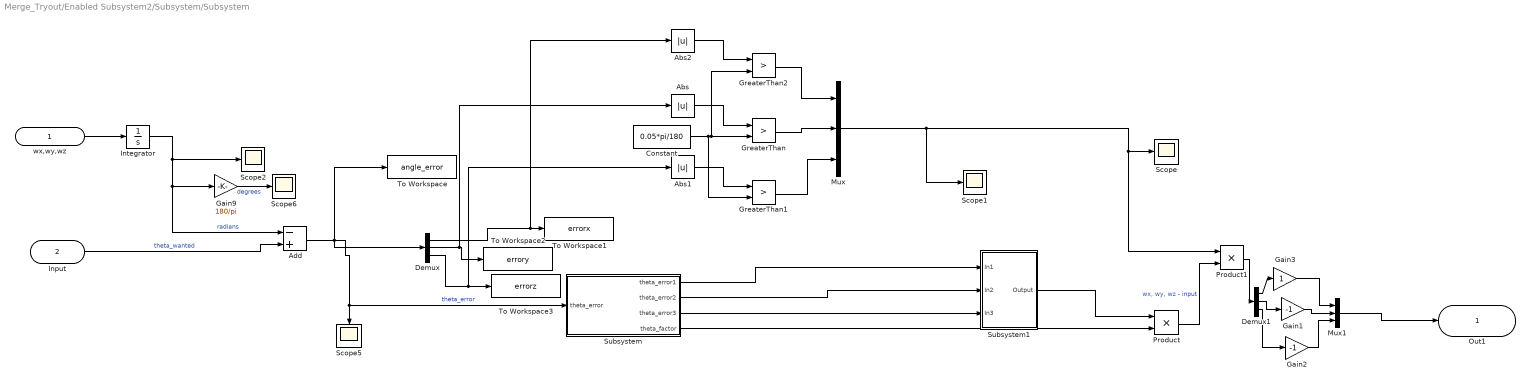
== system Merge_Tryout/Enabled Subsystem2/Subsystem/Subsystem ==
  wx,wy,wz : Inport
  Input : Inport  Port=2
  Abs : Abs
  Abs1 : Abs
  Abs2 : Abs
  Add : Sum  Inputs=-+
  Constant : Constant  Value=0.05*pi/180
  Demux : Demux  Outputs=3
  Demux1 : Demux  Outputs=3
  Gain1 : Gain  Gain=-1
  Gain2 : Gain  Gain=-1
  Gain3 : Gain
  Gain9 : Gain  Gain=180/pi
  GreaterThan : RelationalOperator  Operator=>  OutDataTypeStr=boolean  RndMeth=Simplest
  GreaterThan1 : RelationalOperator  Operator=>  OutDataTypeStr=boolean  RndMeth=Simplest
  GreaterThan2 : RelationalOperator  Operator=>  OutDataTypeStr=boolean  RndMeth=Simplest
  Integrator : Integrator  InitialCondition=[0;0;0]
  Mux : Mux  Inputs=3
  Mux1 : Mux  Inputs=3
  Product : Product
  Product1 : Product
  Scope{,1..2,5..6} (5 alike) : Scope
  Subsystem : Subsystem
  Subsystem1 : Subsystem
  To Workspace : ToWorkspace  VariableName=angle_error  SampleTime=-1
  To Workspace1 : ToWorkspace  VariableName=errorx  SaveFormat=Timeseries  SampleTime=-1
      settings: Save2DSignal=2-D array (concatenate along first dimension)
  To Workspace2 : ToWorkspace  VariableName=errory  SaveFormat=Timeseries  SampleTime=-1
  To Workspace3 : ToWorkspace  VariableName=errorz  SaveFormat=Timeseries  SampleTime=-1
  Out1 : Outport
  wires:
  Integrator/1 -> Add/1, Gain9/1, Scope2/1  "radians"
  Add/1 -> To Workspace/1, Demux/1, Subsystem/1(theta_error), Scope5/1  "theta_error"
  Gain9/1 -> Scope6/1  "degrees"
  Input/1 -> Add/2  "theta_wanted"
  Product/1 -> Product1/2  "wx, wy, wz - input"
  wx,wy,wz/1 -> Integrator/1
  Subsystem/4(theta_factor) -> Product/2
  Demux/2 -> Abs/1, To Workspace2/1
  Demux/3 -> Abs1/1, To Workspace3/1
  Demux/1 -> Abs2/1, To Workspace1/1
  Subsystem/1(theta_error1) -> Subsystem1/1(In1)
  Subsystem/2(theta_error2) -> Subsystem1/2(In2)
  Subsystem/3(theta_error3) -> Subsystem1/3(In3)
  Subsystem1/1(Output) -> Product/1
  Abs/1 -> GreaterThan/1
  Constant/1 -> GreaterThan1/2, GreaterThan2/2, GreaterThan/2
  Abs1/1 -> GreaterThan1/1
  Abs2/1 -> GreaterThan2/1
  GreaterThan2/1 -> Mux/1
  GreaterThan/1 -> Mux/2
  GreaterThan1/1 -> Mux/3
  Mux/1 -> Scope1/1, Scope/1, Product1/1
  Product1/1 -> Demux1/1
  Mux1/1 -> Out1/1
  Demux1/2 -> Gain1/1
  Demux1/3 -> Gain2/1
  Demux1/1 -> Gain3/1
  Gain3/1 -> Mux1/1
  Gain1/1 -> Mux1/2
  Gain2/1 -> Mux1/3

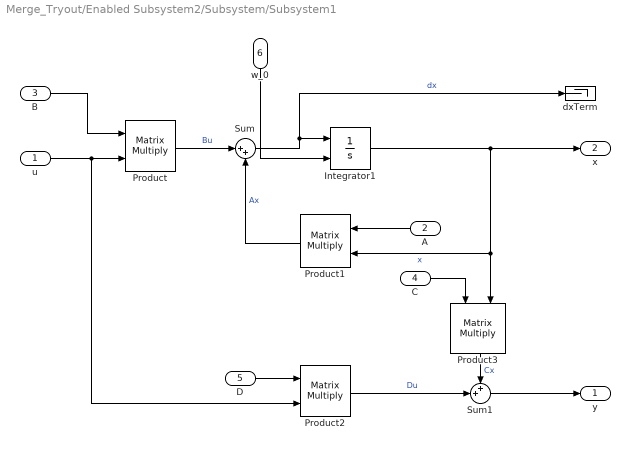
== system Merge_Tryout/Enabled Subsystem2/Subsystem/Subsystem1 ==
  u : Inport
  A : Inport  Port=2
  B : Inport  Port=3
  C : Inport  Port=4
  D : Inport  Port=5
  w_0 : Inport  Port=6
  Integrator1 : Integrator  InitialConditionSource=external  InitialCondition=[0;0;0]
  Product{,1..3} (4 alike) : Product  SCDEnableBlockLinearizationSpecification=on  Multiplication=Matrix(*)
  Sum : Sum  Inputs=|++
  Sum1 : Sum  Inputs=++|
  dxTerm : Terminator
  y : Outport  VectorParamsAs1DForOutWhenUnconnected=off
  x : Outport  Port=2  VectorParamsAs1DForOutWhenUnconnected=off
  wires:
  Sum/1 -> Integrator1/1, dxTerm/1  "dx"
  Product3/1 -> Sum1/1  "Cx"
  Product/1 -> Sum/1  "Bu"
  u/1 -> Product2/2, Product/2
  Product2/1 -> Sum1/2  "Du"
  Integrator1/1 -> x/1, Product1/2, Product3/2  "x"
  A/1 -> Product1/1
  Product1/1 -> Sum/2  "Ax"
  C/1 -> Product3/1
  B/1 -> Product/1
  D/1 -> Product2/1
  Sum1/1 -> y/1
  w_0/1 -> Integrator1/2

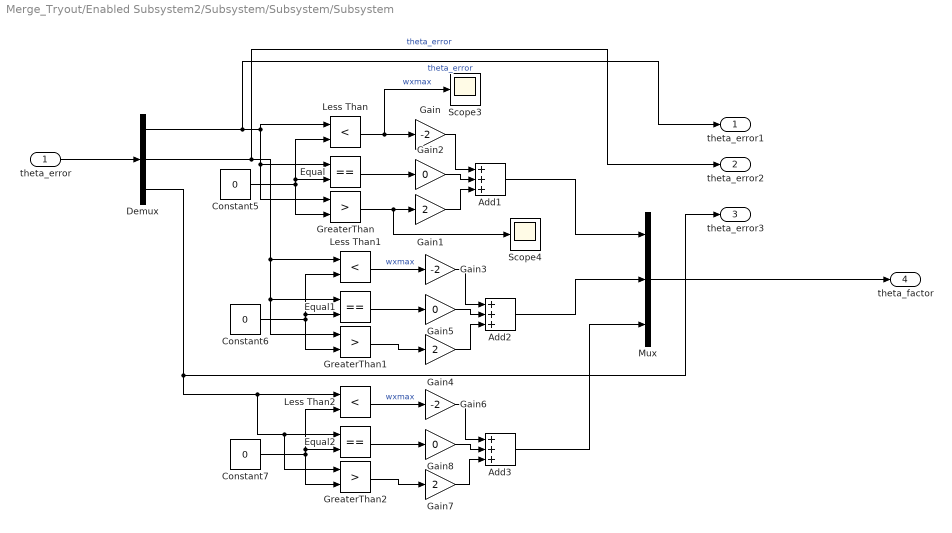
== system Merge_Tryout/Enabled Subsystem2/Subsystem/Subsystem/Subsystem ==
  theta_error : Inport
  Add1 : Sum  Inputs=+++
  Add2 : Sum  Inputs=+++
  Add3 : Sum  Inputs=+++
  Constant5 : Constant  Value=0
  Constant6 : Constant  Value=0
  Constant7 : Constant  Value=0
  Demux : Demux  Outputs=3
  Equal : RelationalOperator  Operator===  OutDataTypeStr=boolean  RndMeth=Simplest
  Equal1 : RelationalOperator  Operator===  OutDataTypeStr=boolean  RndMeth=Simplest
  Equal2 : RelationalOperator  Operator===  OutDataTypeStr=boolean  RndMeth=Simplest
  Gain : Gain  Gain=-2
  Gain1 : Gain  Gain=2
  Gain2 : Gain  Gain=0
  Gain3 : Gain  Gain=-2
  Gain4 : Gain  Gain=2
  Gain5 : Gain  Gain=0
  Gain6 : Gain  Gain=-2
  Gain7 : Gain  Gain=2
  Gain8 : Gain  Gain=0
  GreaterThan : RelationalOperator  Operator=>  OutDataTypeStr=boolean  RndMeth=Simplest
  GreaterThan1 : RelationalOperator  Operator=>  OutDataTypeStr=boolean  RndMeth=Simplest
  GreaterThan2 : RelationalOperator  Operator=>  OutDataTypeStr=boolean  RndMeth=Simplest
  Less Than : RelationalOperator  Operator=<  OutDataTypeStr=boolean  RndMeth=Simplest
  Less Than1 : RelationalOperator  Operator=<  OutDataTypeStr=boolean  RndMeth=Simplest
  Less Than2 : RelationalOperator  Operator=<  OutDataTypeStr=boolean  RndMeth=Simplest
  Mux : Mux  Inputs=3
  Scope3 : Scope
  Scope4 : Scope
  theta_error1 : Outport
  theta_error2 : Outport  Port=2
  theta_error3 : Outport  Port=3
  theta_factor : Outport  Port=4
  wires:
  Add1/1 -> Mux/1
  Constant5/1 -> Equal/2, Less Than/2, GreaterThan/2
  Equal2/1 -> Gain8/1
  Demux/1 -> theta_error1/1, GreaterThan/1, Equal/1, Less Than/1  "theta_error"
  GreaterThan2/1 -> Gain7/1
  Gain1/1 -> Add1/3
  Gain7/1 -> Add3/3
  Less Than1/1 -> Gain3/1  "wxmax"
  Gain6/1 -> Add3/1
  Equal/1 -> Gain2/1
  Gain5/1 -> Add2/2
  Add3/1 -> Mux/3
  GreaterThan/1 -> Scope4/1, Gain1/1
  Constant6/1 -> Equal1/2, Less Than1/2, GreaterThan1/2
  Demux/3 -> theta_error3/1, GreaterThan2/1, Equal2/1, Less Than2/1
  Gain3/1 -> Add2/1
  Constant7/1 -> Equal2/2, Less Than2/2, GreaterThan2/2
  Equal1/1 -> Gain5/1
  Gain8/1 -> Add3/2
  Gain4/1 -> Add2/3
  GreaterThan1/1 -> Gain4/1
  Gain/1 -> Add1/1
  Demux/2 -> theta_error2/1, GreaterThan1/1, Equal1/1, Less Than1/1  "theta_error"
  Gain2/1 -> Add1/2
  Add2/1 -> Mux/2
  Less Than/1 -> Scope3/1, Gain/1  "wxmax"
  Less Than2/1 -> Gain6/1  "wxmax"
  theta_error/1 -> Demux/1
  Mux/1 -> theta_factor/1

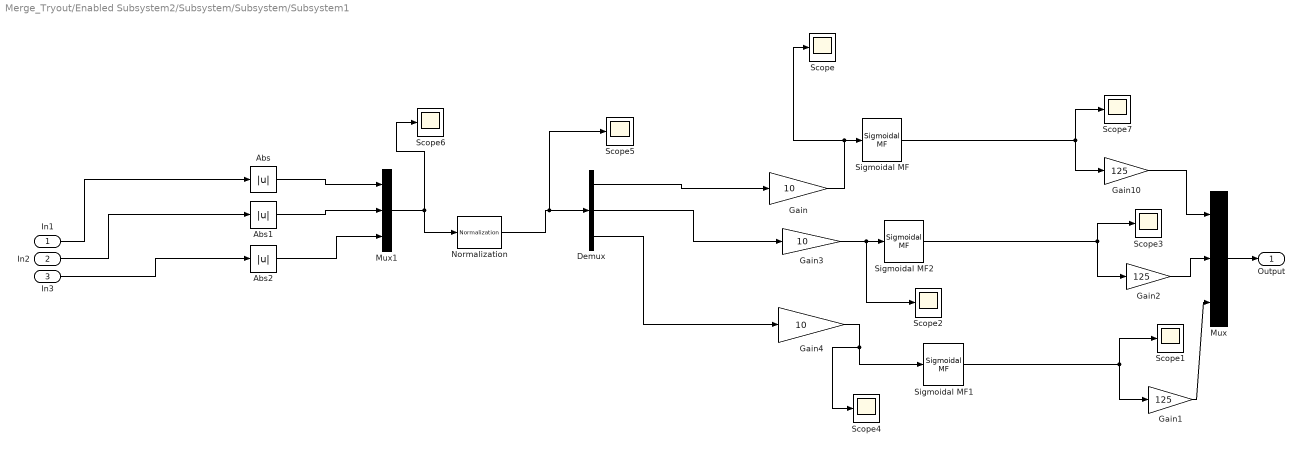
== system Merge_Tryout/Enabled Subsystem2/Subsystem/Subsystem/Subsystem1 ==
  In1 : Inport
  In2 : Inport  Port=2
  In3 : Inport  Port=3
  Abs : Abs
  Abs1 : Abs
  Abs2 : Abs
  Demux : Demux  Outputs=3
  Gain : Gain  Gain=10
  Gain1 : Gain  Gain=125
  Gain10 : Gain  Gain=125
  Gain2 : Gain  Gain=125
  Gain3 : Gain  Gain=10
  Gain4 : Gain  Gain=10
  Mux : Mux  Inputs=3
  Mux1 : Mux  Inputs=3
  Normalization : dspmathops/Normalization  NormType=Squared 2-norm  Bias=1e-10  NormOver=Each column  Dimension=1  roundingMode=Floor  overflowMode=off  accumDataTypeStr=Inherit: Same as product output  accumLastDataTypeStr=Inherit: Same as product output  outputDataTypeStr=Inherit: Same as product output  outputMin=[]  outputMax=[]  outputLastDataTypeStr=Inherit: Same as product output
  Scope{,1..7} (8 alike) : Scope
  Sigmoidal MF : fuzblock/Membership  Functions/Sigmoidal MF  a=10^(-8)  c=1000
      settings: SourceProductBaseCode=FL
  Sigmoidal MF1 : fuzblock/Membership  Functions/Sigmoidal MF  a=10^(-8)  c=1000
      settings: SourceProductBaseCode=FL
  Sigmoidal MF2 : fuzblock/Membership  Functions/Sigmoidal MF  a=10^(-8)  c=1000
      settings: SourceProductBaseCode=FL
  Output : Outport
  wires:
  Gain2/1 -> Mux/2
  Gain10/1 -> Mux/1
  Sigmoidal MF1/1 -> Gain1/1, Scope1/1
  Sigmoidal MF/1 -> Gain10/1, Scope7/1
  Sigmoidal MF2/1 -> Gain2/1, Scope3/1
  Gain/1 -> Scope/1, Sigmoidal MF/1
  Gain1/1 -> Mux/3
  Gain3/1 -> Scope2/1, Sigmoidal MF2/1
  In2/1 -> Abs1/1
  In1/1 -> Abs/1
  In3/1 -> Abs2/1
  Mux/1 -> Output/1
  Abs/1 -> Mux1/1
  Abs1/1 -> Mux1/2
  Gain4/1 -> Scope4/1, Sigmoidal MF1/1
  Abs2/1 -> Mux1/3
  Demux/3 -> Gain4/1
  Demux/1 -> Gain/1
  Demux/2 -> Gain3/1
  Mux1/1 -> Normalization/1, Scope6/1
  Normalization/1 -> Scope5/1, Demux/1
